simulink model "camera_test_model_right"  (R2013a)
settings: Solver=ode3  StartTime=0.0  StopTime=T  FixedStep=t_samples  RelTol=1e-3
values from neighbouring files (symbols this model uses):
  t_samples = 0.1    [wide_trajectory.mat]
undefined symbols (not defined in the file or in its folder): Rec, SDTV, strel
libraries: simulink x4, vrlib x3, visionstatistics x1, visionmorphops x1, visionconversions x1, visionsinks x1
settings Model: Creator=HP  LastModifiedBy=HP

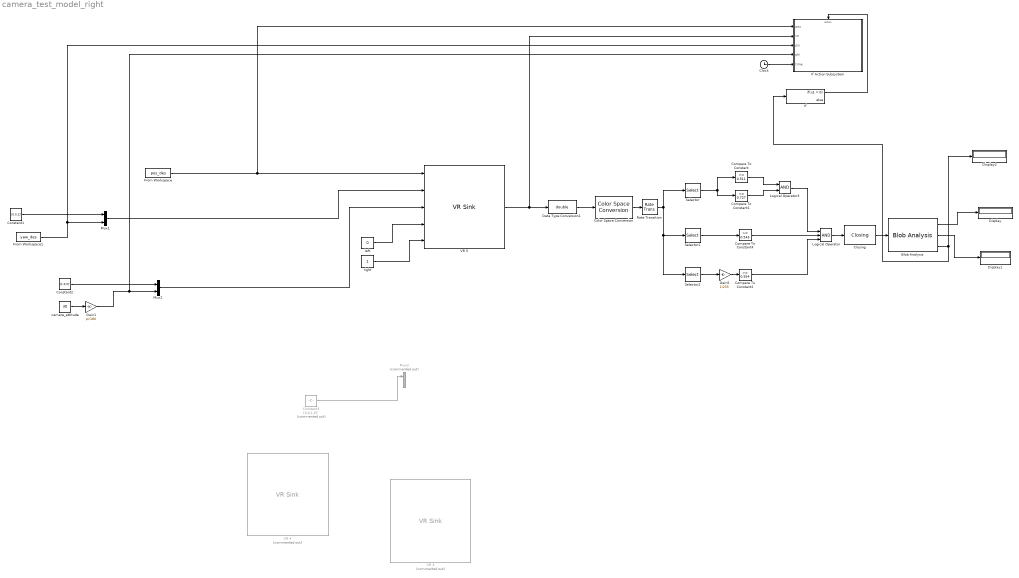
== system camera_test_model_right ==
  Blob Analysis : visionstatistics/Blob Analysis  Tag=vipblks_row_conv  area=on  centroid=on  bBox=off  majorAxis=off  minorAxis=off  angle=off  eccentricity=off  equivDiameterSq=off  extent=off  perimeter=off  maxBlobs=1  warnIfNumBlobsExceeded=on  isCount=on  useMinArea=on  minArea=30  useMaxArea=off  maxArea=intmax('uint32')  excludeBorderBlob=on  outDT=double  isOutVarDim=off  isFill=on  fillValues=-1  conn=8  isLabel=off  outputMode=Binary point scaling  outputWordLength=32  outputFracLength=16  firstCoeffMode=Binary point scaling  firstCoeffWordLength=16  firstCoeffFracLength=14  secondCoeffMode=Binary point scaling  secondCoeffWordLength=32  secondCoeffFracLength=16  accumMode=Binary point scaling  accumWordLength=32  accumFracLength=0  prodOutputMode=Binary point scaling  prodOutputWordLength=32  prodOutputFracLength=16  roundingMode=Floor  overflowMode=off
  Clock : Clock
  Closing : visionmorphops/Closing  nhoodsrc=Specify via dialog  strel=strel('disk',2)
  Color Space Conversion : visionconversions/Color Space  Conversion  conversion=Obsolete  conversionActive=R'G'B' to HSV  wp_str=D65  rec=Rec. 601 (SDTV)  sys=1125/60/2:1  imagePorts=One multidimensional signal
  Compare To Constant : simulink/Logic and Bit Operations/Compare To Constant  relop=>=  const=0.511  OutDataTypeStr=boolean
  Compare To Constant1 : simulink/Logic and Bit Operations/Compare To Constant  relop=<=  const=0.727  OutDataTypeStr=boolean
  Compare To Constant2 : simulink/Logic and Bit Operations/Compare To Constant  relop=>=  const=0.554  OutDataTypeStr=boolean
  Compare To Constant4 : simulink/Logic and Bit Operations/Compare To Constant  relop=>=  const=0.543  OutDataTypeStr=boolean
  Constant1 : Constant  Value=[0,0,1]'
  Constant2 : Constant  Value=[1,0,0]'
  Constant3 : Constant  Commented=on  Value=[0,0,1,0]'
  Data Type Conversion1 : DataTypeConversion  OutDataTypeStr=double
  Display : Display
  Display1 : Display
  Display2 : Display
  From Workspace : FromWorkspace  VariableName=pos_des  SampleTime=0
  From Workspace1 : FromWorkspace  VariableName=yaw_des  SampleTime=0
  Gain1 : Gain  Gain=pi/180
  Gain5 : Gain  Gain=1/255
  If : If  SampleTime=t_samples
  If Action Subsystem : Subsystem  TreatAsAtomicUnit=on
  Logical Operator : Logic  Inputs=3  AllPortsSameDT=off  OutDataTypeStr=boolean
  Logical Operator3 : Logic  AllPortsSameDT=off  OutDataTypeStr=boolean
  Mux1 : Mux  Inputs=2
  Mux2 : Mux  Inputs=2
  Mux3 : Mux  Commented=on  Inputs=2
  Rate Transition : RateTransition
  Selector : Selector  NumberOfDimensions=3  InputPortWidth=3  IndexOptions=Index vector (dialog),Index vector (dialog),Index vector (dialog)  Indices=1:480,1:640,1  OutputSizes=1,1,1
  Selector1 : Selector  NumberOfDimensions=3  InputPortWidth=3  IndexOptions=Index vector (dialog),Index vector (dialog),Index vector (dialog)  Indices=1:480,1:640,2  OutputSizes=1,1,1
  Selector2 : Selector  NumberOfDimensions=3  InputPortWidth=3  IndexOptions=Index vector (dialog),Index vector (dialog),Index vector (dialog)  Indices=1:480,1:640,3  OutputSizes=1,1,1
  VR 3 : vrlib/VR Sink  Commented=on  InstantiateOnLoad=on  SampleTime=t_samples  ViewEnable=on  RemoteChange=off  RemoteView=off  FieldsWritten=TopView.set_bind.1.1.1.logical#TopView.fieldOfView.1.1.1.double#Drone.translation.3.1.1.double#RotationZ.rotation.4.1.1.double#RotationX.rotation.4.1.1.double#left_cam.set_bind.1.1.1.logical#right_cam.set_bind.1.1.1.logical  WorldFileName=texture\LearningSceneBlue.wrl  AutoView=off  VideoDimensions=[480 640]  AllowVariableSize=off  FigureProperties="{'Position', 'Name', 'Viewpoint', 'CameraBound', 'CameraDirection', 'CameraPosition', 'CameraUpVector', 'ZoomFactor', 'Antialiasing', 'Headlight', 'Lighting', 'NavPanel', 'StatusBar', 'ToolBar', 'Textures', 'Transparency', 'Triad', 'Wireframe', 'NavZones', 'NavMode', 'NavSpeed', 'CaptureFileFormat', 'CaptureFileName', 'Record2DCompressMethod', 'Record2DCompressQuality', 'Record2D', 'Record2DFileName', 'Record2DFPS'; [3.0000000000000000e+01   6.0000000000000000e+01   6.4000000000000000e+02   4.8000000000000000e+02], '', 'right_cam', 'on', [0.0000000000000000e+00   0.0000000000000000e+00  -1.0000000000000000e+00], [0.0000000000000000e+00   0.0000000000000000e+00   0.0000000000000000e+00], [0.0000000000000000e+00   1.0000000000000000e+00   0.0000000000000000e+00], [1.0000000000000000e+00], 'on', 'on', 'on', 'none', 'off', 'off', 'on', 'on', 'none', 'off', 'off', 'examine', 'normal', 'tif', '%f_anim_%n.tif', 'auto', [7.5000000000000000e+01], 'off', '***video***', [1.5000000000000000e+01]}"
  VR 4 : vrlib/VR Sink  Commented=on  InstantiateOnLoad=on  SampleTime=t_samples  ViewEnable=on  RemoteChange=off  RemoteView=off  FieldsWritten=Drone.translation.3.1.1.double#RotationZ.rotation.4.1.1.double#RotationX.rotation.4.1.1.double#left_cam.set_bind.1.1.1.logical#right_cam.set_bind.1.1.1.logical  WorldFileName=texture\LearningScene4Wpts.wrl  AutoView=off  VideoDimensions=[480 640]  AllowVariableSize=off  FigureProperties="{'Position', 'Name', 'Viewpoint', 'CameraBound', 'CameraDirection', 'CameraPosition', 'CameraUpVector', 'ZoomFactor', 'Antialiasing', 'Headlight', 'Lighting', 'NavPanel', 'StatusBar', 'ToolBar', 'Textures', 'Transparency', 'Triad', 'Wireframe', 'NavZones', 'NavMode', 'NavSpeed', 'CaptureFileFormat', 'CaptureFileName', 'Record2DCompressMethod', 'Record2DCompressQuality', 'Record2D', 'Record2DFileName', 'Record2DFPS'; [3.0000000000000000e+01   6.0000000000000000e+01   6.4000000000000000e+02   4.8000000000000000e+02], '', 'right_cam', 'on', [0.0000000000000000e+00   0.0000000000000000e+00  -1.0000000000000000e+00], [0.0000000000000000e+00   0.0000000000000000e+00   0.0000000000000000e+00], [0.0000000000000000e+00   1.0000000000000000e+00   0.0000000000000000e+00], [1.0000000000000000e+00], 'on', 'on', 'on', 'none', 'off', 'off', 'on', 'on', 'none', 'off', 'off', 'examine', 'normal', 'tif', '%f_anim_%n.tif', 'auto', [7.5000000000000000e+01], 'off', '***video***', [1.5000000000000000e+01]}"
  "VR 5 " : vrlib/VR Sink  InstantiateOnLoad=on  SampleTime=t_samples  ViewEnable=on  RemoteChange=off  RemoteView=off  FieldsWritten=Drone.translation.3.1.1.double#RotationZ.rotation.4.1.1.double#RotationX.rotation.4.1.1.double#left_cam.set_bind.1.1.1.logical#right_cam.set_bind.1.1.1.logical  WorldFileName=LearningSceneWide.wrl  AutoView=off  VideoDimensions=[480 640]  AllowVariableSize=off  FigureProperties="{'Position', 'Name', 'Viewpoint', 'CameraBound', 'CameraDirection', 'CameraPosition', 'CameraUpVector', 'ZoomFactor', 'Antialiasing', 'Headlight', 'Lighting', 'NavPanel', 'StatusBar', 'ToolBar', 'Textures', 'Transparency', 'Triad', 'Wireframe', 'NavZones', 'NavMode', 'NavSpeed', 'CaptureFileFormat', 'CaptureFileName', 'Record2DCompressMethod', 'Record2DCompressQuality', 'Record2D', 'Record2DFileName', 'Record2DFPS'; [3.0000000000000000e+01   6.0000000000000000e+01   6.4000000000000000e+02   4.8000000000000000e+02], '', 'right_cam', 'on', [0.0000000000000000e+00   0.0000000000000000e+00  -1.0000000000000000e+00], [0.0000000000000000e+00   0.0000000000000000e+00   0.0000000000000000e+00], [0.0000000000000000e+00   1.0000000000000000e+00   0.0000000000000000e+00], [1.0000000000000000e+00], 'on', 'on', 'on', 'none', 'off', 'off', 'on', 'on', 'none', 'off', 'off', 'examine', 'normal', 'tif', '%f_anim_%n.tif', 'auto', [7.5000000000000000e+01], 'off', '***video***', [1.5000000000000000e+01]}"
  camera_attitude : Constant  Value=30
  left : Constant  Value=0  SampleTime=-1
  "right " : Constant
  wires:
  left/1 -> "VR 5 "/4
  "right "/1 -> "VR 5 "/5
  Constant1/1 -> Mux1/1
  From Workspace1/1 -> If Action Subsystem/3(psi), Mux1/2
  Constant2/1 -> Mux2/1
  camera_attitude/1 -> Gain1/1
  Gain1/1 -> If Action Subsystem/4(phi), Mux2/2
  Constant3/1 -> Mux3/1
  Mux1/1 -> "VR 5 "/2
  Mux2/1 -> "VR 5 "/3
  From Workspace/1 -> If Action Subsystem/1(pos), "VR 5 "/1
  "VR 5 "/1 -> If Action Subsystem/2(im), Data Type Conversion1/1
  Color Space Conversion/1 -> Rate Transition/1
  Compare To Constant/1 -> Logical Operator3/1
  Compare To Constant1/1 -> Logical Operator3/2
  Logical Operator3/1 -> Logical Operator/1
  Logical Operator/1 -> Closing/1
  Compare To Constant4/1 -> Logical Operator/2
  Selector/1 -> Compare To Constant1/1, Compare To Constant/1
  Closing/1 -> Blob Analysis/1
  Selector1/1 -> Compare To Constant4/1
  Selector2/1 -> Gain5/1
  Data Type Conversion1/1 -> Color Space Conversion/1
  Rate Transition/1 -> Selector/1, Selector2/1, Selector1/1
  Gain5/1 -> Compare To Constant2/1
  Compare To Constant2/1 -> Logical Operator/3
  Blob Analysis/1 -> Display/1
  Blob Analysis/2 -> Display1/1
  Blob Analysis/3 -> If/1, Display2/1
  If/1 -> If Action Subsystem/Action
  Clock/1 -> If Action Subsystem/5(time)

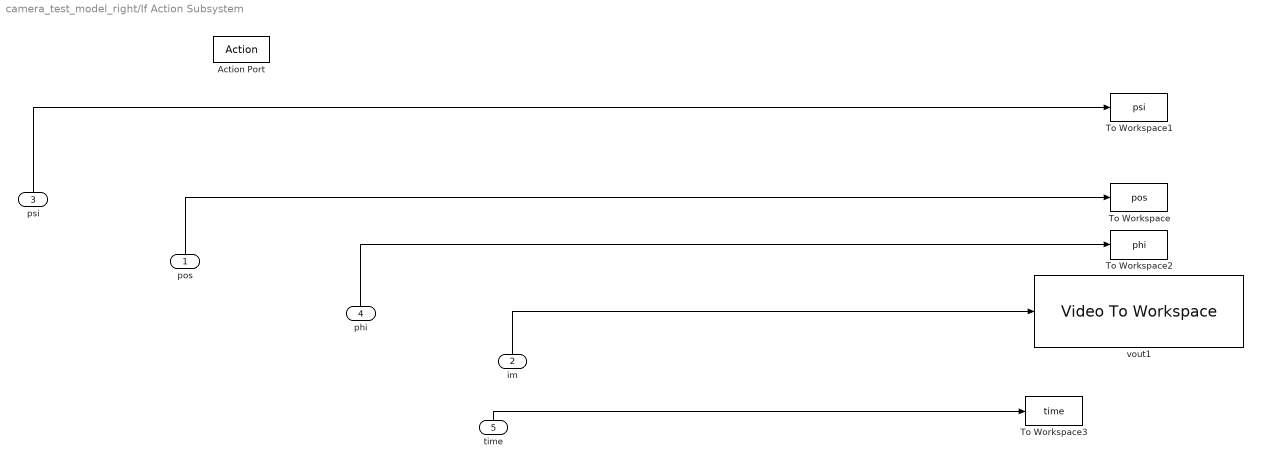
== system camera_test_model_right/If Action Subsystem ==
  pos : Inport
  im : Inport  Port=2
  psi : Inport  Port=3
  phi : Inport  Port=4
  time : Inport  Port=5
  Action Port : ActionPort  ActionType=then
  To Workspace : ToWorkspace  VariableName=pos  SampleTime=t_samples  SaveFormat=Structure
  To Workspace1 : ToWorkspace  VariableName=psi  SampleTime=t_samples  SaveFormat=Structure
  To Workspace2 : ToWorkspace  VariableName=phi  SampleTime=t_samples  SaveFormat=Structure
  To Workspace3 : ToWorkspace  VariableName=time  SampleTime=t_samples  SaveFormat=Structure
  vout1 : visionsinks/Video To Workspace  VariableName=vout_right  NumInputs=1  DataLimit=inf  DecimationFactor=1  LogFi=off  InPortLabels=R|G|B
  wires:
  psi/1 -> To Workspace1/1
  pos/1 -> To Workspace/1
  phi/1 -> To Workspace2/1
  im/1 -> vout1/1
  time/1 -> To Workspace3/1
